simulink model "wheelset_discrete_V5"  (Simulink 7.8)
settings: Solver=FixedStepDiscrete  StartTime=0.0  StopTime=10.0  FixedStep=Delta_t  RelTol=1e-3
values from neighbouring files (symbols this model uses):
  q = [x;y;z;a;b;c;theta_W_R;u_W_R;theta_W_L;u_W_L;u_R_R;x_R_R;u_R_L;x_R_L;]    [environment.m]    (also in kalker_pruebas.m = qn +  0.5 * delta_t * ( dqn + dqn1 ))
undefined symbols (not defined in the file or in its folder): Delta_t
settings Model: Creator=imac  LastModifiedBy=aitor
settings DebuggingCC: FcnCallInpInsideContextMsg=Use local settings

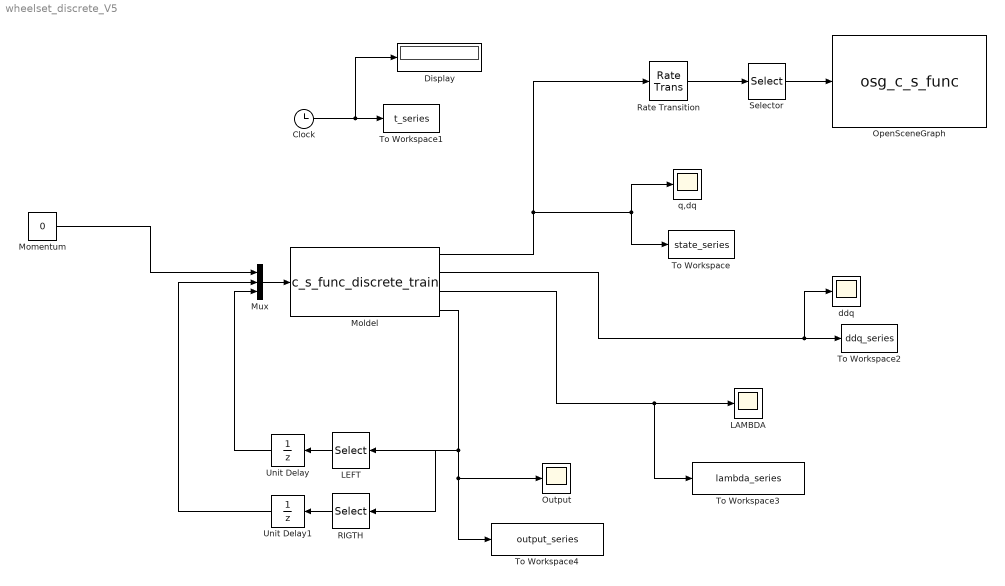
== system wheelset_discrete_V5 ==
  Clock : Clock
  Display : Display
  LAMBDA : Scope
      settings: YMin=-1  YMax=6  SaveName=ScopeData2  SampleInput=on
  LEFT : Selector  InputPortWidth=26  IndexOptions=Index vector (dialog)  Indices=21:1:23  OutputSizes=1
  Moldel : S-Function  FunctionName=c_s_func_discrete_train  Parameters=q dq param Delta_t  EnableBusSupport=off
      mask Type: S-function: mycsfunc
      mask Description: This is a S-function that does the continuous state space system.
      mask Display: disp('[M , Phi_q''] [ddq]\n[Phi_q , 0] [lambda]\n=\n [Q ] \n   [gamma] ');
  Momentum : Constant  Value=0
  Mux : Mux  Inputs=3
  OpenSceneGraph : S-Function  FunctionName=osg_c_s_func  EnableBusSupport=off
  Output : Scope
      settings: YMin=0  YMax=6000  SaveName=ScopeData3  SampleInput=on
  RIGTH : Selector  InputPortWidth=26  IndexOptions=Index vector (dialog)  Indices=24:1:26  OutputSizes=1
  Rate Transition : RateTransition  OutPortSampleTime=0.04
  Selector : Selector  InputPortWidth=2*length(q)  IndexOptions=Index vector (dialog)  Indices=1:1:length(q)  OutputSizes=1
  To Workspace : ToWorkspace  VariableName=state_series  SampleTime=Delta_t  SaveFormat=Array
  To Workspace1 : ToWorkspace  VariableName=t_series  SampleTime=Delta_t  SaveFormat=Array
  To Workspace2 : ToWorkspace  VariableName=ddq_series  SampleTime=Delta_t  SaveFormat=Array
  To Workspace3 : ToWorkspace  VariableName=lambda_series  SampleTime=Delta_t  SaveFormat=Array
  To Workspace4 : ToWorkspace  VariableName=output_series  SampleTime=Delta_t  SaveFormat=Array
  Unit Delay : UnitDelay  SampleTime=-1
  Unit Delay1 : UnitDelay  SampleTime=-1
  ddq : Scope
      settings: YMin=-500  YMax=300  SampleInput=on
  q,dq : Scope
      settings: YMin=-0.03  YMax=0.17  SampleInput=on  SampleTime=Delta_t
  wires:
  Clock/1 -> To Workspace1/1, Display/1
  Moldel/1 -> q,dq/1, To Workspace/1, Rate Transition/1
  Moldel/2 -> ddq/1, To Workspace2/1
  Moldel/3 -> To Workspace3/1, LAMBDA/1
  Moldel/4 -> Output/1, To Workspace4/1, LEFT/1, RIGTH/1
  Selector/1 -> OpenSceneGraph/1
  Rate Transition/1 -> Selector/1
  Mux/1 -> Moldel/1
  Momentum/1 -> Mux/1
  RIGTH/1 -> Unit Delay1/1
  Unit Delay/1 -> Mux/3
  Unit Delay1/1 -> Mux/2
  LEFT/1 -> Unit Delay/1
